simulink model "vector_projection"  (R2014b)
settings: Solver=FixedStepDiscrete  StartTime=3600  StopTime=4200  FixedStep=0.01  RelTol=1e-3
libraries: util_quat_lib x2
settings Model: Creator=Jim Kaidy  LastModifiedBy=mstewart
settings DataIOCC: SignalLoggingSaveFormat=ModelDataLogs
settings DebuggingCC: AlgebraicLoopMsg=error  ArtificialAlgebraicLoopMsg=error  UnderspecifiedInitializationDetection=Classic  MergeDetectMultiDrivingBlocksExec=none

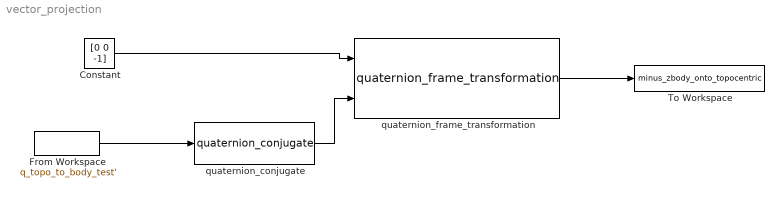
== system vector_projection ==
  Constant : Constant  Value=[0 0 -1]
  From Workspace : FromWorkspace  VariableName=q_topo_to_body_test'  SampleTime=0.01  Interpolate=off  OutputAfterFinalValue=Holding final value
  To Workspace : ToWorkspace  VariableName=minus_zbody_onto_topocentric  SaveFormat=Timeseries  SampleTime=-1
  quaternion_conjugate : util_quat_lib/quaternion_conjugate  SystemSampleTime=-1
  quaternion_frame_transformation : util_quat_lib/quaternion_frame_transformation  SystemSampleTime=-1
  wires:
  From Workspace/1 -> quaternion_conjugate/1
  quaternion_conjugate/1 -> quaternion_frame_transformation/2
  Constant/1 -> quaternion_frame_transformation/1
  quaternion_frame_transformation/1 -> To Workspace/1
